simulink model "prob2"  (R2024a)
settings: Solver=VariableStepAuto  StartTime=0.0  StopTime=10.0  MaxStep=0.01  RelTol=1e-3
settings Model: Creator=yeseo  LastModifiedBy=yeseo

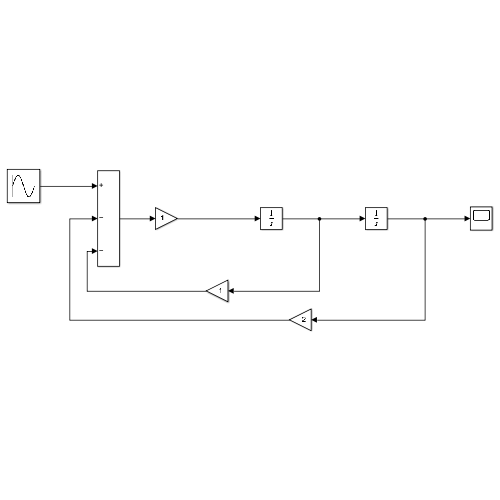
[thumbnail: Simulink's stored preview of the top-level diagram]
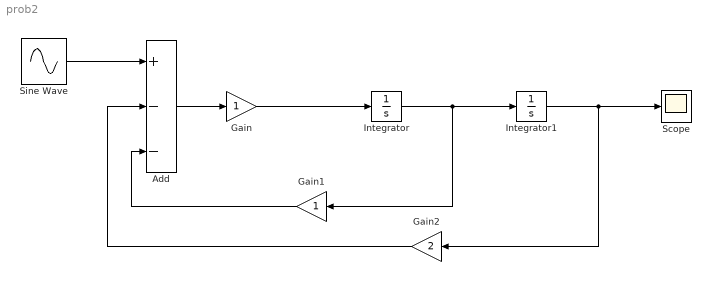
== system prob2 ==
  Add : Sum  Inputs=+--
  Gain : Gain
  Gain1 : Gain
  Gain2 : Gain  Gain=2
  Integrator : Integrator
  Integrator1 : Integrator
  Scope : Scope
  Sine Wave : Sin  Frequency=5  SampleTime=0
  wires:
  Sine Wave/1 -> Add/1
  Add/1 -> Gain/1
  Integrator1/1 -> Scope/1, Gain2/1
  Integrator/1 -> Gain1/1, Integrator1/1
  Gain/1 -> Integrator/1
  Gain1/1 -> Add/3
  Gain2/1 -> Add/2
